simulink model "sec2_3"  (R2018b)
settings: Solver=VariableStepAuto  StartTime=0.0  StopTime=300  MaxStep=0.01  RelTol=1e-3
undefined symbols (not defined in the file): a, b, c, d
settings Model: Creator=buddyugwumba1  LastModifiedBy=buddyugwumba1

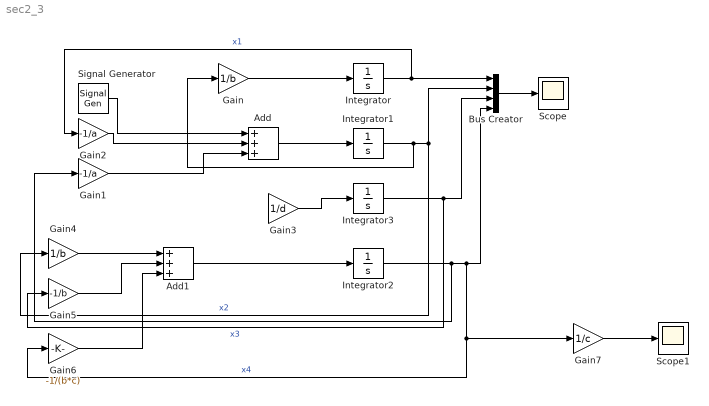
== system sec2_3 ==
  Add : Sum  Inputs=+++
  Add1 : Sum  Inputs=+++
  Bus Creator : BusCreator  Inputs=4
  Gain : Gain  Gain=1/b
  Gain1 : Gain  Gain=-1/a
  Gain2 : Gain  Gain=-1/a
  Gain3 : Gain  Gain=1/d
  Gain4 : Gain  Gain=1/b
  Gain5 : Gain  Gain=-1/b
  Gain6 : Gain  Gain=-1/(b*c)
  Gain7 : Gain  Gain=1/c
  Integrator{,1..3} (4 alike) : Integrator
  Scope : Scope
  Scope1 : Scope
  Signal Generator : SignalGenerator  Frequency=50  Units=rad/sec
  wires:
  Bus Creator/1 -> Scope/1
  Integrator/1 -> Gain2/1, Bus Creator/1  "x1"
  Gain/1 -> Integrator/1
  Add/1 -> Integrator1/1
  Integrator1/1 -> Gain/1, Gain4/1, Bus Creator/2  "x2"
  Gain1/1 -> Add/3
  Gain2/1 -> Add/2
  Signal Generator/1 -> Add/1
  Gain3/1 -> Integrator3/1
  Integrator3/1 -> Gain5/1, Bus Creator/3  "x3"
  Gain4/1 -> Add1/1
  Gain5/1 -> Add1/2
  Gain6/1 -> Add1/3
  Add1/1 -> Integrator2/1
  Integrator2/1 -> Gain1/1, Gain7/1, Gain6/1, Bus Creator/4  "x4"
  Gain7/1 -> Scope1/1
